simulink model "InverseKinematics"  (R2022a)
settings: Solver=ode4  StartTime=0.0  StopTime=Inf  FixedStep=1/500  RelTol=1e-3
libraries: quarc_library x2, simulink_extras x1
settings Model: ExtModeTrigDuration=10000  Creator=fvranes  LastModifiedBy=lgonzalez
settings SolverCC: AlgebraicLoopSolver=TrustRegion
settings DataIOCC: ReturnWorkspaceOutputs=off
settings DebuggingCC: UnderspecifiedInitializationDetection=Classic  MergeDetectMultiDrivingBlocksExec=none  UnconnectedInputMsg=warning  UnconnectedOutputMsg=warning  UnconnectedLineMsg=warning
settings ModelReferenceCC: PropagateSignalLabelsOutOfModel=off
settings SFSimCC: CustomCodeUndefinedFunction=UseInterfaceOnly

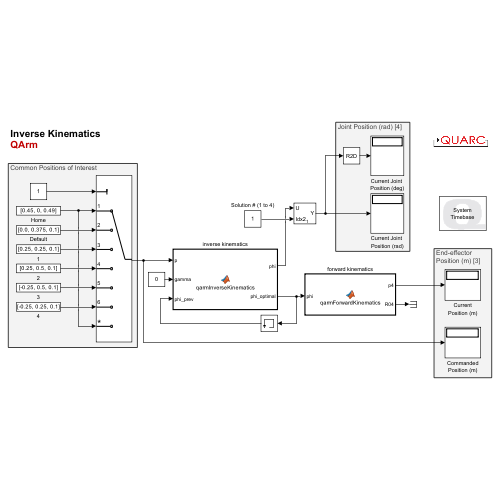
[thumbnail: Simulink's stored preview of the top-level diagram]
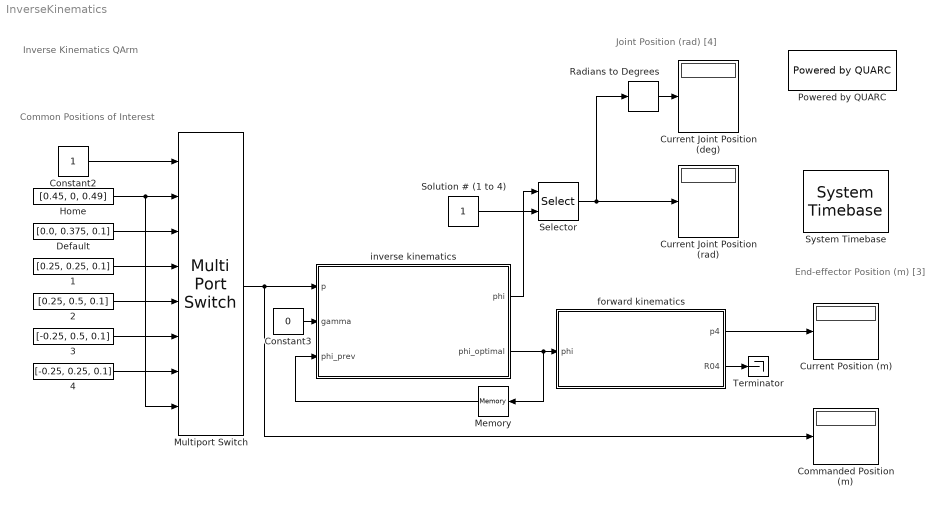
== system InverseKinematics ==
  note: End-effector
      | Position (m) [3]
  note: Common Positions of Interest
  note: Joint Position (rad) [4]
  note: Inverse Kinematics
      | QArm
  1 : Constant  Value=[0.25, 0.25, 0.1]
  2 : Constant  Value=[0.25, 0.5, 0.1]
  3 : Constant  Value=[-0.25, 0.5, 0.1]
  4 : Constant  Value=[-0.25, 0.25, 0.1]
  Commanded Position (m) : Display
  Constant2 : Constant
  Constant3 : Constant  Value=0
  Current Position (m) : Display
  Current Joint Position (deg) : Display
  Current Joint Position (rad) : Display
  Default : Constant  Value=[0.0, 0.375, 0.1]
  Home : Constant  Value=[0.45, 0, 0.49]
  Memory : Memory  InitialCondition=[0 0 0 0]
  Multiport Switch : MultiPortSwitch  Inputs=6  DataPortForDefault=Additional data port  SaturateOnIntegerOverflow=off  InputSameDT=off
  Powered by QUARC : quarc_library/Logos/Powered by QUARC
  Radians to Degrees : simulink_extras/Transformations/Radians to Degrees
  Selector : Selector  NumberOfDimensions=2  InputPortWidth=3  IndexOptions=Select all,Index vector (port)  Indices=[1 3],1  OutputSizes=1,1
  Solution # (1 to 4) : Constant
  System Timebase : quarc_library/Advanced/Timing/System Timebase  stop_on_overrun=off
      settings: SourceProductName=QUARC Targets
  Terminator : Terminator
  forward kinematics : MATLAB Function  TreatAsAtomicUnit=on
  inverse kinematics : MATLAB Function  TreatAsAtomicUnit=on
  wires:
  forward kinematics/2(R04) -> Terminator/1
  forward kinematics/1(p4) -> Current Position (m)/1
  Multiport Switch/1 -> Commanded Position (m)/1, inverse kinematics/1(p)
  Constant3/1 -> inverse kinematics/2(gamma)
  Home/1 -> Multiport Switch/8, Multiport Switch/2
  Default/1 -> Multiport Switch/3
  Constant2/1 -> Multiport Switch/1
  1/1 -> Multiport Switch/4
  2/1 -> Multiport Switch/5
  3/1 -> Multiport Switch/6
  4/1 -> Multiport Switch/7
  inverse kinematics/2(phi_optimal) -> forward kinematics/1(phi), Memory/1
  Memory/1 -> inverse kinematics/3(phi_prev)
  Radians to Degrees/1 -> Current Joint Position (deg)/1
  inverse kinematics/1(phi) -> Selector/1
  Selector/1 -> Radians to Degrees/1, Current Joint Position (rad)/1
  Solution # (1 to 4)/1 -> Selector/2

== matlab function InverseKinematics/forward kinematics ==
  data: phi input; p4 output; R04 output
function [p4, R04] = qarmForwardKinematics(phi)

%% QUANSER_ARM_FPK
% v 4.0 - 4th June 2020

% REFERENCE: 
% Chapter 3. Forward Kinematics
% Robot Dynamics and Control 
% Spong, Vidyasagar
% 1989

% INPUTS:
% phi     : Alternate joint angles vector 4 x 1

% OUTPUTS:
% p4      : End-effector frame {4} position vector expressed in base frame {0}
% R04     : rotation matrix from end-effector frame {4} to base frame {0}

%% Manipulator parameters:
L1 = 0.1400;
L2 = 0.3500;
L3 = 0.0500;
L4 = 0.2500;
L5 = 0.1500;

%% Alternate parameters
l1 = ;
l2 = ;
l3 = ;
beta = ;

%% From phi space to theta space 
theta = phi;
theta(1) = phi(1);
theta(2) = phi(2);
theta(3) = phi(3);
theta(4) = phi(4);

%% Transformation matrices for all frames:

% T{i-1}{i} = quanser_arm_DH(  a, alpha,  d,     theta );
        T01 = quanser_arm_DH(  0,     0,  0,         0 );
        T12 = quanser_arm_DH(  0,     0,  0,         0 );
        T23 = quanser_arm_DH(  0,     0,  0,         0 );
        T34 = quanser_arm_DH(  0,     0,  0,         0 );

        T02 = ;
        T03 = ;
        T04 = ;

%% Position of end-effector Transformation

% Extract the Position vector 
p4 = ;

% Extract the Rotation matrix
R04 = ;

end

function T = quanser_arm_DH(a,alpha,d,theta)

%% QUANSER_ARM_DH
% v 1.0 - 26th March 2019

% REFERENCE: 
% Chapter 3. Forward and Inverse Kinematics
% Robot Modeling and Control 
% Spong, Hutchinson, Vidyasagar
% 2006

% INPUTS:
% a       :   translation  : along : x_{i}   : from : z_{i-1} : to : z_{i}
% alpha   :      rotation  : about : x_{i}   : from : z_{i-1} : to : z_{i}
% d       :   translation  : along : z_{i-1} : from : x_{i-1} : to : x_{i}
% theta   :      rotation  : about : z_{i-1} : from : x_{i-1} : to : x_{i}
% NOTE: Standard DH Parameters

% OUTPUTS:
% T       : transformation                   : from :     {i} : to : {i-1}

%%
% Rotation Transformation about z axis by theta
T_R_z = ;
     
% Translation Transformation along z axis by d
T_T_z = ;

% Translation Transformation along x axis by a
T_T_x = ;

% Rotation Transformation about x axis by alpha
T_R_x = ;

% For a transformation FROM frame {i} TO frame {i-1}:
% rotate about z
% then translate along z, 
% then translate along x, 
% then rotate about x, 

T = ;

end

== matlab function InverseKinematics/inverse kinematics ==
  data: phi output; p input; gamma input; phi_optimal output; phi_prev input
function [phi, phi_optimal]  = qarmInverseKinematics(p, gamma, phi_prev)

%% QUANSER_ARM_IPK
% v 4.0 - 4th June 2020

% REFERENCE: 
% Chapter 4. Inverse Kinematics
% Robot Dynamics and Control 
% Spong, Vidyasagar
% 1989

% INPUTS:
% p        : end-effector position vector expressed in base frame {0}
% gamma    : wrist rotation angle gamma

% OUTPUTS:
% phi_optimal : Best solution depending on phi_prev
% phi         : All four Inverse Kinematics solutions as a 4x4 matrix. 
%               Each col is a solution.

%% Manipulator parameters:
L1 = 0.1400;
L2 = 0.3500;
L3 = 0.0500;
L4 = 0.2500;
L5 = 0.1500;
beta = ;

%% Alternate parameters
lambda1 = ;
lambda2 = ;
lambda3 = ;

%% Initialization
theta = zeros(4, 4);
phi = zeros(4, 4);

%% Joint angle 2 and 3: 
% Equations:
    % lambda2 cos(theta2) + (-lambda3) sin(theta2 + theta3) = sqrt(x^2 + y^2)
    %   A     cos( 2    ) +     C      sin(   2   +    3  ) =    D
    
    % lambda2 sin(theta2) - (-lambda3) cos(theta2 + theta3) = lambda1 - z
    %   A     sin( 2    ) -     C      cos(   2   +    3  ) =    H

% Solution:
    A = ;
    C = ;
    H = ;
    D1 = ;
    D2 = ;
    F = ;

    theta(3,1) = 2*atan2( C + sqrt(C^2 - F^2) , F );
	theta(3,2) = 2*atan2( C - sqrt(C^2 - F^2) , F );
    theta(3,3) = theta(3,1);
	theta(3,4) = theta(3,2);

    M = ;
    N = ;
    cos_term = ;
    sin_term = ;
    theta(2,1) = atan2(sin_term, cos_term);

    M = ;
    N = ;
    cos_term = ;
    sin_term = ;
    theta(2,2) = atan2(sin_term, cos_term);

    M = ;
    N = ;
    cos_term = ;
    sin_term = ;
    theta(2,3) = atan2(sin_term, cos_term);

    M = ;
    N = ;
    cos_term = ;
    sin_term = ;
    theta(2,4) = atan2(sin_term, cos_term);


%% Joint angle 1:
% Equation:
    % y / x = tan(theta1);

% Solution
    theta(1,1) = ;
    theta(1,2) = ;
    theta(1,3) = ;
    theta(1,4) = ;
    
%% Remap theta back to phi
phi(1,:) = ;
phi(2,:) = ;
phi(3,:) = ;
phi(4,:) = ;

phi = mod(phi + pi, 2*pi) - pi;

phi_optimal = phi(:,1);
if (norm(phi_optimal - phi_prev) > norm(phi(:,2) - phi_prev)) || (check_joint_limits(phi_optimal))
    phi_optimal = phi(:,2);
end
if (norm(phi_optimal - phi_prev) > norm(phi(:,3) - phi_prev)) || (check_joint_limits(phi_optimal))
    phi_optimal = phi(:,3);
end
if (norm(phi_optimal - phi_prev) > norm(phi(:,4) - phi_prev)) || (check_joint_limits(phi_optimal))
    phi_optimal = phi(:,4);
end
if (check_joint_limits(phi_optimal))
    phi_optimal = [0;0;0;0];
end

end

function flag = check_joint_limits(phi)
    flag = 0;
    if phi(1) > 170*pi/180 || phi(1) < -170*pi/180 ...
        || phi(2) > 80*pi/180 || phi(2) < -80*pi/180 ...
        || phi(3) > 75*pi/180 || phi(3) < -95*pi/180 ...
        || phi(4) > 160*pi/180 || phi(4) < -160*pi/180
    flag = 1;
    end
end
